simulink model "MPCtest"  (R2021b)
settings: Solver=VariableStepAuto  StartTime=0.0  StopTime=30  RelTol=1e-3
libraries: dspnetwork x2, sldrtlib x1
settings Model: Creator=Kuorun Liu  LastModifiedBy=Kuorun Liu

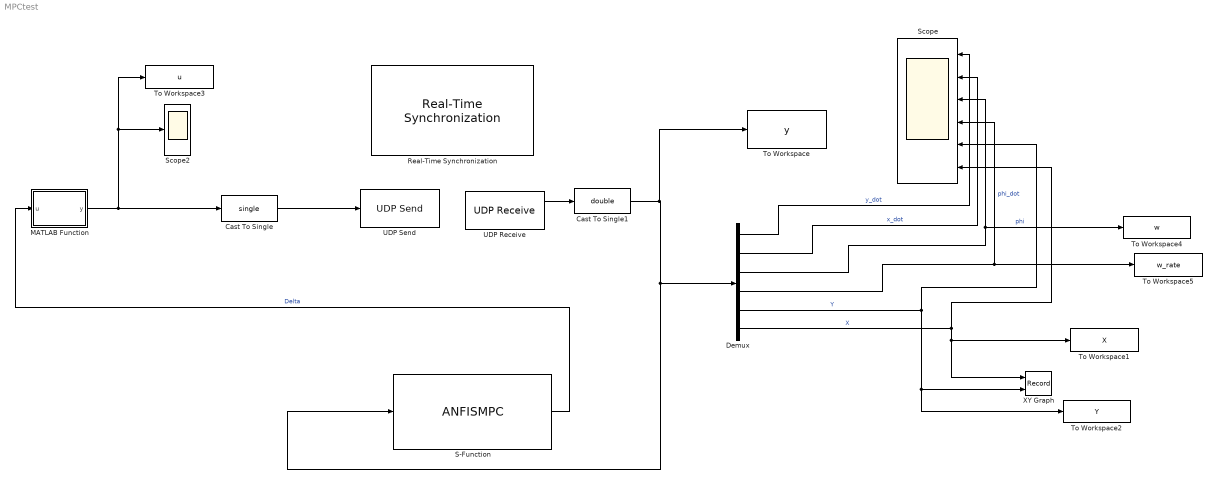
== system MPCtest ==
  Cast To Single : DataTypeConversion  OutDataTypeStr=single
  Cast To Single1 : DataTypeConversion  OutDataTypeStr=double
  Demux : Demux  Outputs=6
  MATLAB Function : MATLAB Function  TreatAsAtomicUnit=on
  Real-Time Synchronization : sldrtlib/Real-Time Synchronization  SampleTime=0.0005  MaxMissedTicks=100000  ShowMissedTicks=off  YieldWhenWaiting=off
  S-Function : S-Function  FunctionName=ANFISMPC  SFunctionDeploymentMode=off  EnableBusSupport=off
  Scope : Scope  NumInputPorts=6
  Scope2 : Scope
  To Workspace : ToWorkspace  VariableName=y  SampleTime=-1
  To Workspace1 : ToWorkspace  VariableName=X  SampleTime=-1
      settings: Save2DSignal=2-D array (concatenate along first dimension)
  To Workspace2 : ToWorkspace  VariableName=Y  SampleTime=-1
      settings: Save2DSignal=2-D array (concatenate along first dimension)
  To Workspace3 : ToWorkspace  VariableName=u  SampleTime=-1
  To Workspace4 : ToWorkspace  VariableName=w  SampleTime=-1
      settings: Save2DSignal=2-D array (concatenate along first dimension)
  To Workspace5 : ToWorkspace  VariableName=w_rate  SampleTime=-1
      settings: Save2DSignal=2-D array (concatenate along first dimension)
  UDP Receive : dspnetwork/UDP Receive  localURL='0.0.0.0'  localPort=2241  remoteURL='0.0.0.0'  remotePort=-1  recvBufferSize=8192  dims=6  signalDatatype=single  isComplex=off  isVarSize=off  showBlockingTime=off  blockingTime=0  sampletime=0.0005  blockPlatform=[]
  UDP Send : dspnetwork/UDP Send  remoteURL='127.0.0.1'  remotePort=2240  localURL='0.0.0.0'  localPortSource=Automatically determine  localPort=-1  sendBufferSize=8192  sampletime=-1  blockPlatform=[]  separateLengthPort=0
  XY Graph : Record  Filename=C:\Users\Kuorun Liu\Desktop\修改\Result plot\plot41.xlsx  FileSettingsInternal="{\"entries\":[{\"content\":{\"excelSettings\":{\"content\":{},\"type\":\"Streamout.ExcelSettings\"}},\"type\":\"Streamout.FileSettingStorage\",\"uuid\":\"e5c6256b-bb7c-4b6f-bf2e-8a0e1984a6b5\"}],\"packageUris\":[\"http://schema.mathworks.com/mf0/streamout_blocks/R2020a\"],\"version\":\"1.0\"}"  Layout=[1 1]  SignalsInternal="{\"entries\":[{\"content\":{\"signals\":[{\"content\":{\"blockPath\":[\"MPCtest/XY Graph\"],\"channel\":[],\"dimensions\":[1,1],\"domain\":\"MPCtest/XY Graph\",\"lineColor\":\"#a2142f\",\"plots\":[1],\"port\":1,\"sid\":[\"\"],\"signalID\":13128,\"signalName\":\"X\"},\"type\":\"RecordBlkView.Signal\",\"uuid\":\"224e1e8f-8e04-4f45-9161-e10f9fedb0df\"},{\"content\":{\"blockPath\":[\"MPCtest/XY Graph\"],\"channel\":[],\"dimensions\":[1,1],\"domain\":\"MPCtest/XY Graph\",\"lineColor\":\"#139fff\",\"plots\":[1],\"port\":2,\"sid\":[\"\"],\"signalID\":13132,\"signalName\":\"Y\"},\"type\":\"RecordBlkView.Signal\",\"uuid\":\"4d283771-560e-45a1-b378-b7829419e64f\"}]},\"type\":\"RecordBlkView.InputSignals\",\"uuid\":\"57993c47-fb93-4fa5-848e-4079e213795e\"}],\"packageUris\":[\"http://schema.mathworks.com/mf0/streamout_blocks/R2020a\"],\"version\":\"1.0\"}"  VisualizationBindings="{\"xyplotplugin\":{\"info\":[{\"series\":[{\"bindingParametersList\":[{\"parameter\":\"X-Axis\",\"signalID\":13128,\"signalName\":\"X\"},{\"parameter\":\"Y-Axis\",\"signalID\":13132,\"signalName\":\"Y\"}],\"seriesID\":729}],\"subplotID\":1}]}}"  CompatibilityTag=XY
  wires:
  UDP Receive/1 -> Cast To Single1/1
  Demux/1 -> Scope/1  "y_dot"
  Demux/2 -> Scope/2  "x_dot"
  Demux/3 -> To Workspace4/1, Scope/3  "phi"
  Demux/4 -> Scope/4, To Workspace5/1  "phi_dot"
  Demux/5 -> Scope/5, XY Graph/2, To Workspace2/1  "Y"
  Demux/6 -> Scope/6, XY Graph/1, To Workspace1/1  "X"
  S-Function/1 -> MATLAB Function/1(u)  "Delta"
  MATLAB Function/1(y) -> To Workspace3/1, Scope2/1, Cast To Single/1
  Cast To Single/1 -> UDP Send/1
  Cast To Single1/1 -> S-Function/1, Demux/1, To Workspace/1

== matlab function MPCtest/MATLAB Function ==
  data: u input; y output
function y = fcn(u)
%y=1.6372*u;
y=2*u;
